simulink model "ACC_hybrid_average_staliro"  (R2021a)
settings: Solver=FixedStepAuto  StartTime=0.0  StopTime=T  FixedStep=Ts  RelTol=1e-3
undefined symbols (not defined in the file): amax_ego, amin_ego, D_default, isTerminate, t_gap, Ts, use_MPC, v0_ego, v0_lead, v_set, x0_ego, x0_lead
libraries: simulink x5, rllib x1, mpcadaslib x1
settings Model: OrderedModelArguments=off  Creator=The MathWorks, Inc.  LastModifiedBy=ldy
settings DataIOCC: ExternalInput=in_lead  ReturnWorkspaceOutputs=off
settings DebuggingCC: SFMachineParentedDataDiag=warning  ArithmeticOperatorsInVariantConditions=warning
settings SFSimCC: SimUseLocalCustomCode=off  CustomCodeUndefinedFunction=UseInterfaceOnly
settings RTWCC: RTWUseLocalCustomCode=off
settings CodeAppCC: StateflowObjectComments=on

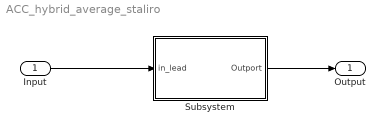
== system ACC_hybrid_average_staliro ==
  Input : Inport
  Subsystem : Subsystem
  Output : Outport
  wires:
  Input/1 -> Subsystem/1(in_lead)
  Subsystem/1(Outport) -> Output/1

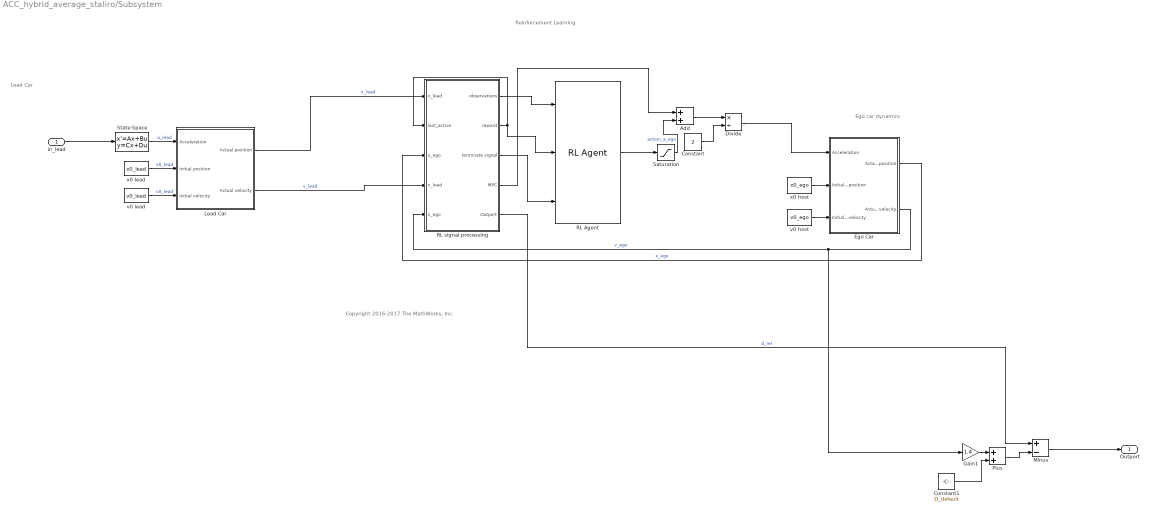
== system ACC_hybrid_average_staliro/Subsystem ==
  note: Ego car dynamics
  note: Reinforcement Learning
  note: Lead Car
  note: Copyright 2016-2017 The MathWorks, Inc.
  in_lead : Inport
  Add : Sum
  Constant : Constant  Value=2
  Constant1 : Constant  Value=D_default
  Divide : Product  Inputs=*/
  Ego Car : Subsystem
  Gain1 : Gain  Gain=1.4
  Lead Car : Subsystem
  Minus : Sum  Inputs=+-
  Plus : Sum
  RL Agent : rllib/RL Agent  Agent=agent  ExternalActionAsInput=off  ProvideCumRwd=off  TreatAsDirectFeedthrough=on
  "RL signal processing " : Subsystem
  Saturation : Saturate  UpperLimit=amax_ego  LowerLimit=amin_ego
  State-Space : StateSpace  A=-10  B=10  D=0  InitialCondition=0
  v0 host : Constant  Value=v0_ego  SampleTime=Ts
  v0 lead : Constant  Value=v0_lead  SampleTime=Ts
  x0 host : Constant  Value=x0_ego  SampleTime=Ts
  x0 lead : Constant  Value=x0_lead  SampleTime=Ts
  Outport : Outport
  wires:
  "RL signal processing "/5(Outport) -> Minus/1  "d_rel"
  v0 host/1 -> Ego Car/3(Initial velocity)
  "RL signal processing "/2(reward) -> RL Agent/2, "RL signal processing "/2(last_action)
  Ego Car/1(Actaul position) -> "RL signal processing "/3(x_ego)  "x_ego"
  State-Space/1 -> Lead Car/1(Acceleration)  "a_lead"
  in_lead/1 -> State-Space/1
  x0 host/1 -> Ego Car/2(Initial position)
  v0 lead/1 -> Lead Car/3(Initial velocity)  "v0_lead"
  Lead Car/1(Actual position) -> "RL signal processing "/1(x_lead)  "x_lead"
  "RL signal processing "/4(MPC) -> Add/1
  Saturation/1 -> Add/2  "action_a_ego"
  Ego Car/2(Actual velocity) -> Gain1/1, "RL signal processing "/5(v_ego)  "v_ego"
  Lead Car/2(Actual velocity) -> "RL signal processing "/4(v_lead)  "v_lead"
  x0 lead/1 -> Lead Car/2(Initial position)  "x0_lead"
  "RL signal processing "/3(terminate signal) -> RL Agent/3
  Divide/1 -> Ego Car/1(Acceleration)
  "RL signal processing "/1(observations) -> RL Agent/1
  Minus/1 -> Outport/1
  Plus/1 -> Minus/2
  Constant1/1 -> Plus/2
  RL Agent/1 -> Saturation/1
  Constant/1 -> Divide/2
  Add/1 -> Divide/1
  Gain1/1 -> Plus/1

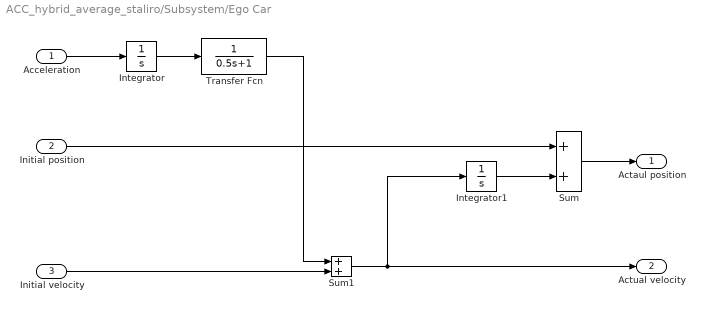
== system ACC_hybrid_average_staliro/Subsystem/Ego Car ==
  Acceleration : Inport
  Initial position : Inport  Port=2
  Initial velocity : Inport  Port=3
  Integrator : Integrator
  Integrator1 : Integrator
  Sum : Sum
  Sum1 : Sum
  Transfer Fcn : TransferFcn  Denominator=[0.5 1]
  Actaul position : Outport  VectorParamsAs1DForOutWhenUnconnected=off
  Actual velocity : Outport  Port=2  VectorParamsAs1DForOutWhenUnconnected=off
  wires:
  Sum1/1 -> Integrator1/1, Actual velocity/1
  Initial velocity/1 -> Sum1/2
  Sum/1 -> Actaul position/1
  Transfer Fcn/1 -> Sum1/1
  Integrator/1 -> Transfer Fcn/1
  Acceleration/1 -> Integrator/1
  Initial position/1 -> Sum/1
  Integrator1/1 -> Sum/2

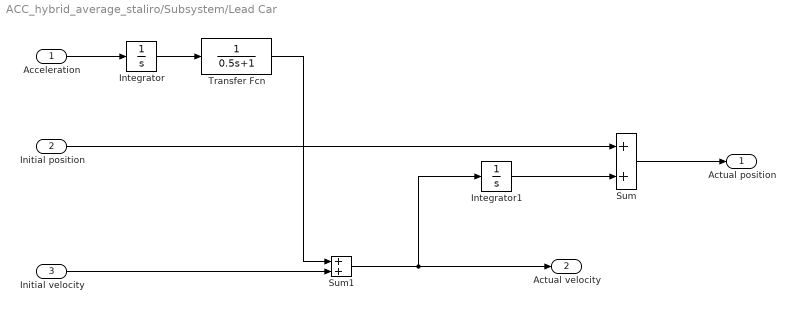
== system ACC_hybrid_average_staliro/Subsystem/Lead Car ==
  Acceleration : Inport
  Initial position : Inport  Port=2
  Initial velocity : Inport  Port=3
  Integrator : Integrator
  Integrator1 : Integrator
  Sum : Sum
  Sum1 : Sum
  Transfer Fcn : TransferFcn  Denominator=[0.5 1]
  Actual position : Outport  VectorParamsAs1DForOutWhenUnconnected=off
  Actual velocity : Outport  Port=2  VectorParamsAs1DForOutWhenUnconnected=off
  wires:
  Transfer Fcn/1 -> Sum1/1
  Initial velocity/1 -> Sum1/2
  Sum/1 -> Actual position/1
  Integrator/1 -> Transfer Fcn/1
  Sum1/1 -> Integrator1/1, Actual velocity/1
  Acceleration/1 -> Integrator/1
  Initial position/1 -> Sum/1
  Integrator1/1 -> Sum/2

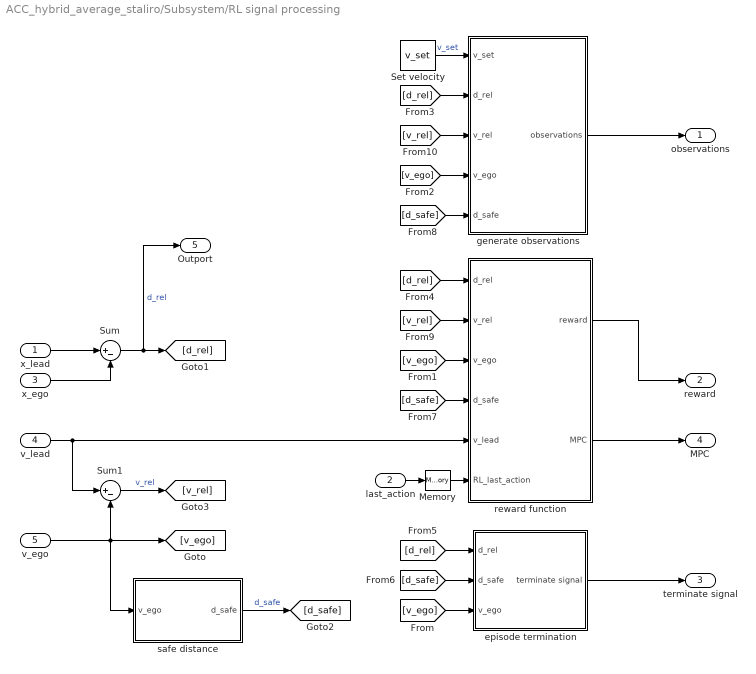
== system ACC_hybrid_average_staliro/Subsystem/RL signal processing  ==
  x_lead : Inport
  last_action : Inport  Port=2
  x_ego : Inport  Port=3
  v_lead : Inport  Port=4
  v_ego : Inport  Port=5
  Memory : Memory
  Set velocity : Constant  Value=v_set  SampleTime=Ts
  Sum : Sum  Inputs=|+-
  Sum1 : Sum  Inputs=|+-
  episode termination : Subsystem
  generate observations : Subsystem
  reward function : Subsystem
  safe distance : Subsystem
  observations : Outport
  reward : Outport  Port=2
  terminate signal : Outport  Port=3
  MPC : Outport  Port=4
  Outport : Outport  Port=5
  wires:
  Sum/1 -> Outport/1, [d_rel]  "d_rel"
  Memory/1 -> reward function/6(RL_last_action)
  v_lead/1 -> Sum1/1, reward function/5(v_lead)
  Set velocity/1 -> generate observations/1(v_set)  "v_set"
  v_ego/1 -> safe distance/1(v_ego), Sum1/2, [v_ego]
  Sum1/1 -> [v_rel]  "v_rel"
  safe distance/1(d_safe) -> [d_safe]  "d_safe"
  generate observations/1(observations) -> observations/1
  reward function/1(reward) -> reward/1
  x_ego/1 -> Sum/2
  x_lead/1 -> Sum/1
  episode termination/1(terminate signal) -> terminate signal/1
  last_action/1 -> Memory/1
  [v_ego] -> episode termination/3(v_ego)
  [v_ego] -> reward function/3(v_ego)
  [v_ego] -> generate observations/4(v_ego)
  [d_rel] -> generate observations/2(d_rel)
  [d_rel] -> reward function/1(d_rel)
  [d_rel] -> episode termination/1(d_rel)
  [d_safe] -> episode termination/2(d_safe)
  [d_safe] -> reward function/4(d_safe)
  [d_safe] -> generate observations/5(d_safe)
  [v_rel] -> reward function/2(v_rel)
  [v_rel] -> generate observations/3(v_rel)
  reward function/2(MPC) -> MPC/1

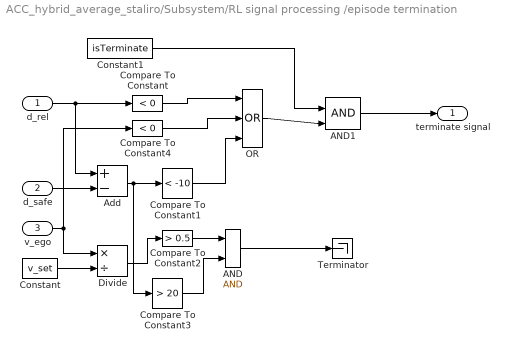
== system ACC_hybrid_average_staliro/Subsystem/RL signal processing /episode termination ==
  d_rel : Inport
  d_safe : Inport  Port=2
  v_ego : Inport  Port=3
  AND : Logic  IconShape=distinctive  AllPortsSameDT=off  OutDataTypeStr=boolean
  AND1 : Logic  IconShape=distinctive  AllPortsSameDT=off  OutDataTypeStr=boolean
  Add : Sum  Inputs=+-
  Compare To Constant : simulink/Logic and Bit Operations/Compare To Constant  relop=<  const=0  OutDataTypeStr=boolean
  Compare To Constant1 : simulink/Logic and Bit Operations/Compare To Constant  relop=<  const=-10  OutDataTypeStr=boolean
  Compare To Constant2 : simulink/Logic and Bit Operations/Compare To Constant  relop=>  const=0.5  OutDataTypeStr=boolean
  Compare To Constant3 : simulink/Logic and Bit Operations/Compare To Constant  relop=>  const=20  OutDataTypeStr=boolean
  Compare To Constant4 : simulink/Logic and Bit Operations/Compare To Constant  relop=<  const=0  OutDataTypeStr=boolean
  Constant : Constant  Value=v_set
  Constant1 : Constant  Value=isTerminate
  Divide : Product  Inputs=*/
  OR : Logic  Operator=OR  Inputs=3  IconShape=distinctive  AllPortsSameDT=off  OutDataTypeStr=boolean
  Terminator : Terminator
  terminate signal : Outport
  wires:
  d_rel/1 -> Compare To Constant/1, Add/1
  Compare To Constant1/1 -> OR/3
  Add/1 -> Compare To Constant1/1, Compare To Constant3/1
  d_safe/1 -> Add/2
  Constant/1 -> Divide/2
  v_ego/1 -> Compare To Constant4/1, Divide/1
  Divide/1 -> Compare To Constant2/1
  Compare To Constant2/1 -> AND/1
  AND/1 -> Terminator/1
  Compare To Constant3/1 -> AND/2
  Compare To Constant/1 -> OR/1
  Compare To Constant4/1 -> OR/2
  OR/1 -> AND1/2
  AND1/1 -> terminate signal/1
  Constant1/1 -> AND1/1

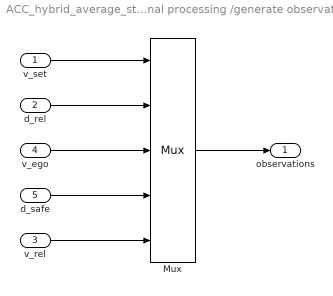
== system ACC_hybrid_average_staliro/Subsystem/RL signal processing /generate observations ==
  v_set : Inport
  d_rel : Inport  Port=2
  v_rel : Inport  Port=3
  v_ego : Inport  Port=4
  d_safe : Inport  Port=5
  Mux : Mux  Inputs=5
  observations : Outport
  wires:
  v_ego/1 -> Mux/3
  v_set/1 -> Mux/1
  Mux/1 -> observations/1
  d_safe/1 -> Mux/4
  v_rel/1 -> Mux/5
  d_rel/1 -> Mux/2

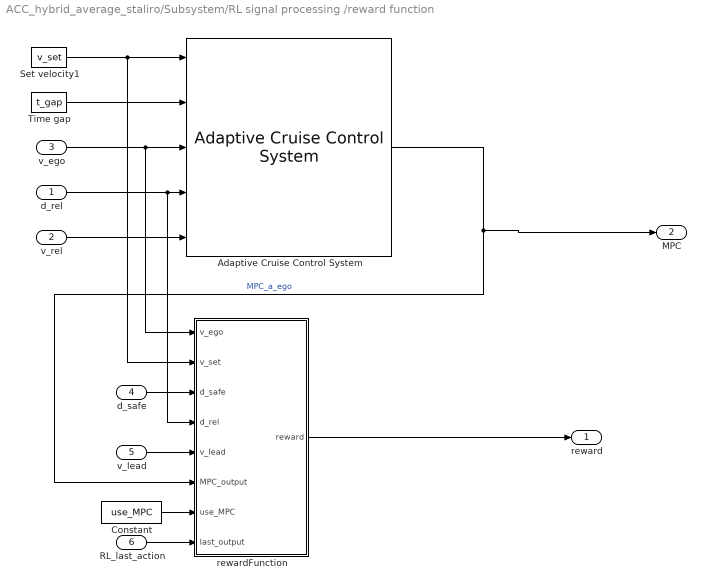
== system ACC_hybrid_average_staliro/Subsystem/RL signal processing /reward function ==
  d_rel : Inport
  v_rel : Inport  Port=2
  v_ego : Inport  Port=3
  d_safe : Inport  Port=4
  v_lead : Inport  Port=5
  RL_last_action : Inport  Port=6
  Adaptive Cruise Control System : mpcadaslib/Adaptive Cruise Control System  EgoModel=tf(1,[0.5,1,0])  InitialEgoVelocity=v0_ego  DefaultSpacing=D_default  MaxVelocity=vmax_ego  MinAcceleration=amin_ego  amin_ext=off  MaxAcceleration=amax_ego  amax_ext=off  Ts=Ts  PredictionHorizon=50  ControllerBehavior=0.500  suboptimal=off  maxiter=10  datatypeopt=double  optmode=off  trackmode=off
  Constant : Constant  Value=use_MPC
  Set velocity1 : Constant  Value=v_set  SampleTime=Ts
  Time gap : Constant  Value=t_gap  SampleTime=Ts
  rewardFunction : MATLAB Function  TreatAsAtomicUnit=on
  reward : Outport
  MPC : Outport  Port=2
  wires:
  v_rel/1 -> Adaptive Cruise Control System/5
  Time gap/1 -> Adaptive Cruise Control System/2
  Set velocity1/1 -> rewardFunction/2(v_set), Adaptive Cruise Control System/1
  d_rel/1 -> rewardFunction/4(d_rel), Adaptive Cruise Control System/4
  v_ego/1 -> rewardFunction/1(v_ego), Adaptive Cruise Control System/3
  Adaptive Cruise Control System/1 -> MPC/1, rewardFunction/6(MPC_output)  "MPC_a_ego"
  rewardFunction/1(reward) -> reward/1
  d_safe/1 -> rewardFunction/3(d_safe)
  v_lead/1 -> rewardFunction/5(v_lead)
  Constant/1 -> rewardFunction/7(use_MPC)
  RL_last_action/1 -> rewardFunction/8(last_output)

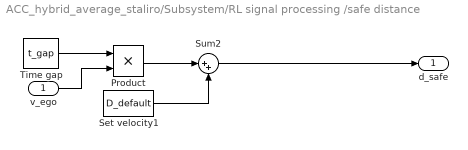
== system ACC_hybrid_average_staliro/Subsystem/RL signal processing /safe distance ==
  v_ego : Inport
  Product : Product
  Set velocity1 : Constant  Value=D_default  SampleTime=Ts
  Sum2 : Sum  Inputs=|++
  Time gap : Constant  Value=t_gap  SampleTime=Ts
  d_safe : Outport
  wires:
  Time gap/1 -> Product/1
  Sum2/1 -> d_safe/1
  v_ego/1 -> Product/2
  Product/1 -> Sum2/1
  Set velocity1/1 -> Sum2/2

== matlab function ACC_hybrid_average_staliro/Subsystem/RL signal processing /reward function/rewardFunction ==
  data: v_ego input; reward output; v_set input; d_safe input; d_rel input; v_lead input; MPC_output input; use_MPC input; last_output input
function reward = fcn(v_ego, v_set, d_safe, d_rel, v_lead, MPC_output, use_MPC, last_output)


% If the relative distance is less than the safe distance, 
% the ego car tracks the minimum of the lead car velocity and driver-set velocity

d_safe = d_safe + 1;

if d_rel <= d_safe
    v_error = v_ego - min(v_set, v_lead);
else
    v_error = v_ego - v_set;
end

if v_error^2 < 0.25
    M_t = 1;
else
    M_t = 0;
end

% reward = -(0.1*v_error^2 + RL_last_1^2) + M_t;

if d_rel< d_safe
    neg_reward = -100*tanh(d_safe-d_rel);
else
    neg_reward = 0;
end


reward = 2*exp(-abs(v_error/10)) + neg_reward - 0.1*abs(last_output/10) + M_t;
